simulink model "nonlinear_simulation_minitvc_v3"  (R2024b)
settings: Solver=ode15s  StartTime=0.0  StopTime=30.0  RelTol=1e-3
values from neighbouring files (symbols this model uses):
  K_hov0 = lqr(sys_red, Q_red, R)    [linear_controller_compute_no_integ.m]
  K_pos = lqr(sys_hor, Q_pos, R_pos)    [linear_controller_compute_no_integ.m]
settings Model: Creator=yoonj  LastModifiedBy=yh583
settings SolverCC: MaxConsecutiveMinStep=2

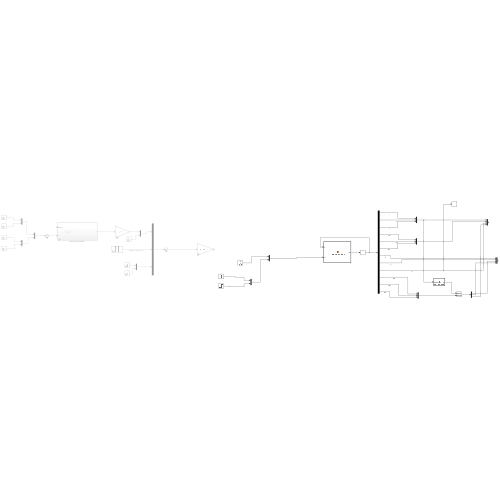
[thumbnail: Simulink's stored preview of the top-level diagram]
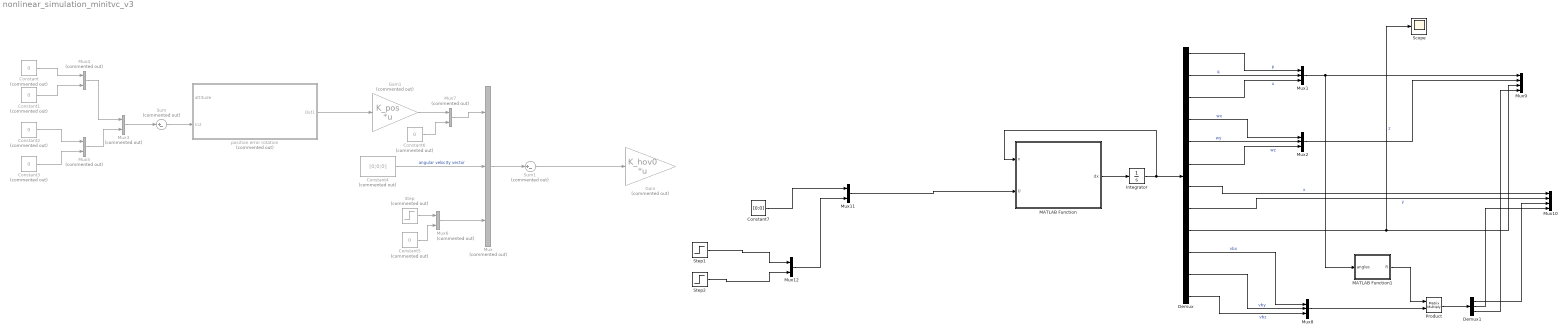
== system nonlinear_simulation_minitvc_v3 ==
  Constant{,1..3,5..6} (6 alike) : Constant  Commented=on  Value=0
  Constant4 : Constant  Commented=on  Value=[0;0;0]  VectorParams1D=off
  Constant7 : Constant  Value=[0;0]  VectorParams1D=off
  Demux : Demux  Outputs=12
  Demux1 : Demux  Outputs=3
  Gain : Gain  Commented=on  Gain=K_hov0  Multiplication=Matrix(K*u)
  Gain1 : Gain  Commented=on  Gain=K_pos  Multiplication=Matrix(K*u)
  Integrator : Integrator  InitialCondition=[0;0;0;0;0;0;0;0;0.01;0;0;0]
  MATLAB Function : MATLAB Function  TreatAsAtomicUnit=on
  MATLAB Function1 : MATLAB Function  TreatAsAtomicUnit=on
  Mux : Mux  Commented=on  Inputs=3
  Mux1 : Mux  Inputs=3
  Mux10 : Mux
  Mux11 : Mux  Inputs=2
  Mux12 : Mux  Inputs=2
  Mux2 : Mux  Inputs=3
  Mux{3..7} (5 alike) : Mux  Commented=on  Inputs=2
  Mux8 : Mux  Inputs=3
  Mux9 : Mux
  Product : Product  Multiplication=Matrix(*)
  Scope : Scope
  Step : Step  Commented=on  SampleTime=0
  Step1 : Step  After=61.6  SampleTime=0
  Step2 : Step  After=61.6  SampleTime=0
  Sum : Sum  Commented=on  Inputs=|+-
  Sum1 : Sum  Commented=on  Inputs=|+-
  position error rotation : Subsystem  Commented=on
  wires:
  MATLAB Function/1(dx) -> Integrator/1
  Integrator/1 -> Demux/1, MATLAB Function/1(x)
  Sum/1 -> position error rotation/2(In2)
  position error rotation/1(Out1) -> Gain1/1
  Mux3/1 -> Sum/1
  Constant/1 -> Mux4/1
  Constant1/1 -> Mux4/2
  Mux4/1 -> Mux3/1
  Constant2/1 -> Mux5/1
  Constant3/1 -> Mux5/2
  Mux5/1 -> Mux3/2
  Sum1/1 -> Gain/1
  Mux/1 -> Sum1/1
  Constant4/1 -> Mux/2  "angular velocity vector"
  Mux6/1 -> Mux/3
  Step/1 -> Mux6/1
  Constant5/1 -> Mux6/2
  Gain1/1 -> Mux7/1
  Mux7/1 -> Mux/1
  Constant6/1 -> Mux7/2
  Demux/2 -> Mux1/2  "q"
  Demux/1 -> Mux1/1  "p"
  Demux/3 -> Mux1/3  "u"
  Demux/4 -> Mux2/1  "wx"
  Demux/5 -> Mux2/2  "wy"
  Demux/6 -> Mux2/3  "wz"
  Demux/10 -> Mux8/1  "vbx"
  Demux/11 -> Mux8/2  "vby"
  Demux/12 -> Mux8/3  "vbz"
  Mux1/1 -> MATLAB Function1/1(angles), Mux9/1
  Mux2/1 -> Mux9/2
  Demux/9 -> Scope/1, Mux9/3  "z"
  MATLAB Function1/1(R) -> Product/1
  Mux8/1 -> Product/2
  Product/1 -> Demux1/1
  Demux1/3 -> Mux9/4
  Demux/7 -> Mux10/1  "x"
  Demux/8 -> Mux10/2  "y"
  Demux1/1 -> Mux10/3
  Demux1/2 -> Mux10/4
  Mux11/1 -> MATLAB Function/2(U)
  Step1/1 -> Mux12/1
  Step2/1 -> Mux12/2
  Mux12/1 -> Mux11/2
  Constant7/1 -> Mux11/1

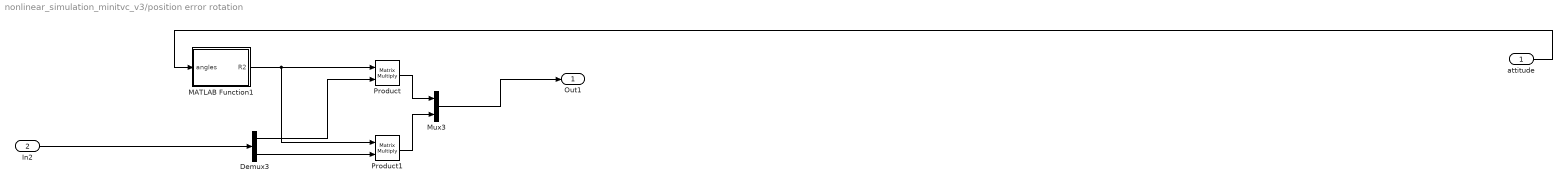
== system nonlinear_simulation_minitvc_v3/position error rotation ==
  attitude : Inport
  In2 : Inport  Port=2
  Demux3 : Demux  Outputs=2
  MATLAB Function1 : MATLAB Function  TreatAsAtomicUnit=on
  Mux3 : Mux  Inputs=2
  Product : Product  Multiplication=Matrix(*)
  Product1 : Product  Multiplication=Matrix(*)
  Out1 : Outport
  wires:
  In2/1 -> Demux3/1
  attitude/1 -> MATLAB Function1/1(angles)
  Demux3/2 -> Product1/2
  MATLAB Function1/1(R2) -> Product1/1, Product/1
  Mux3/1 -> Out1/1
  Demux3/1 -> Product/2
  Product1/1 -> Mux3/2
  Product/1 -> Mux3/1

== matlab function nonlinear_simulation_minitvc_v3/MATLAB Function ==
  data: x input; dx output; U input
function dx = nonlinear_dynamics(x, U)
    % States
    p = x(1); 
    q = x(2);
    u = x(3);

    wx = x(4);
    wy = x(5);
    wz = x(6);

    px = x(7);
    py = x(8);
    pz = x(9);

    vx = x(10);
    vy = x(11);
    vz = x(12);


    a1 = U(1); a2 = U(2); wt1 = U(3); wt2 = U(4);

    % Drone Constants
    Kt = 0.2;      % N / (1/s^2)
    Jx = 0.01;          % Kg * m^2
    Jy = 0.01;    % Kg * m^2
    Jz = 0.003;    % Kg * m^2
    m = 0.75;           % Kg
    g = 9.807;          % m/s^2
    a = 0.1;            % m
    b = 0.1;            % m 
    Km = 0.00016;          % Moment arm constant

    dp = wx + (wz*cos(p)*sin(q))/cos(q) + (wy*sin(p)*sin(q))/cos(q);
    dq = wy*cos(p) - wz*sin(p);
    du = (wz*cos(p))/cos(q) + (wy*sin(p))/cos(q); 

    dwx = -(Jz*wy*wz - Jy*wy*wz - Km*wt1^2*cos(a1)*sin(a2) + Km*wt2^2*cos(a1)*sin(a2) + Kt*a*wt1^2*sin(a1) + Kt*a*wt2^2*sin(a1))/Jx;
    dwy = -(Km*wt1^2*sin(a1) - Km*wt2^2*sin(a1) + Jx*wx*wz - Jz*wx*wz + Kt*a*wt1^2*cos(a1)*sin(a2) + Kt*a*wt2^2*cos(a1)*sin(a2))/Jy;
    dwz = (Km*cos(a1)*cos(a2)*wt1^2 - Km*cos(a1)*cos(a2)*wt2^2 + Jx*wx*wy - Jy*wx*wy)/Jz;
    
    dpx = vz*(sin(p)*sin(u) + cos(p)*cos(u)*sin(q)) - vy*(cos(p)*sin(u) - cos(u)*sin(p)*sin(q)) + vx*cos(q)*cos(u);
    dpy = vy*(cos(p)*cos(u) + sin(p)*sin(q)*sin(u)) - vz*(cos(u)*sin(p) - cos(p)*sin(q)*sin(u)) + vx*cos(q)*sin(u);
    dpz = vz*cos(p)*cos(q) - vx*sin(q) + vy*cos(q)*sin(p);
    
    dvx = (g*m*sin(q) + Kt*cos(a1)*sin(a2)*(wt1^2 + wt2^2))/m;
    dvy = -(Kt*sin(a1)*(wt1^2 + wt2^2) + g*m*cos(q)*sin(p))/m;
    dvz = (Kt*cos(a1)*cos(a2)*(wt1^2 + wt2^2) - g*m*cos(p)*cos(q))/m;
    
    % if the toal force in the body-z direction is larger han gravity (dvz)
    % or the drone already is in the air (pz >0), return all derivatives
    %if (dvz > 0 || pz  > 0 )
        % return the derivatives
        %dx = [dp; dq; du; dwx; dwy; dwz; dpx; dpy; dpz; dvx; dvy; dvz ];
    
    %else 
        %dx = [dp; dq; du; dwx; dwy; dwz; 0;0;0;0;0;0];

    %end

    dx = [dp; dq; du; dwx; dwy; dwz; dpx; dpy; dpz; dvx; dvy; dvz ];
end

== matlab function nonlinear_simulation_minitvc_v3/position error rotation/MATLAB Function1 ==
  data: angles input; R2 output
function R2 = world_to_body(angles)
u = angles(3);

R2 = [ cos(u) sin(u);
       -sin(u) cos(u)];

== matlab function nonlinear_simulation_minitvc_v3/MATLAB Function1 ==
  data: angles input; R output
function R = body_to_world(angles)
p = angles(1);
q = angles(2);
u = angles(3);

R = [cos(q)*cos(u), sin(p)*sin(q)*cos(u)-cos(p)*sin(u), cos(p)*sin(q)*cos(u)+sin(p)*sin(u) ;
     cos(q)*sin(u), sin(p)*sin(q)*sin(u)+cos(p)*cos(u), cos(p)*sin(q)*sin(u)-sin(p)*cos(u) ;
     -sin(q),       sin(p)*cos(q),                      cos(p)*cos(q)                     ];
